simulink model "DFADAS2_SenFus_v1_201204RC_training_210115"  (R2018b)
settings: Solver=FixedStepDiscrete  StartTime=0.0  StopTime=inf  FixedStep=0.002  RelTol=1e-3  EnableMultiTasking=on
PreLoadFcn:
  | RTWConfigurationCB('preloadfcn', bdroot);
libraries: canmsglib x108, simulink x48, canfdmsglib x12
(part 17 of 28)

== system DFADAS2_SenFus_v1_201204RC_training_210115/Signal Input (Input)/Signal Input (50ms) (Input50)/Rear Right Radar(S1) Objects Information (RRRdr)/S0 Data Frame Read/Enabled Subsystem/M4ObjInfo1 ==
  msg : Inport
  MValue : Inport  Port=2
  RemainderCnt : Inport  Port=3
  obj_num : Inport  Port=4
  Add3 : Sum
  Bus Creator1 : BusCreator  Inputs=24
  Bus Creator2 : BusCreator  Inputs=24
  Constant : Constant  Value=9
  Data Type Conversion{,1..3} (4 alike) : DataTypeConversion  OutDataTypeStr=uint16
  Data Type Conversion5 : DataTypeConversion  OutDataTypeStr=int16
  Demux : Demux  Outputs=24
  Demux1 : Demux  Outputs=24
  If : If  NumInputs=3  IfExpression=u1 == 1  ElseIfExpressions=u2 == 0 & u3 == 1  ShowElse=off
  If Action Subsystem1 : Subsystem  TreatAsAtomicUnit=on
  If Action Subsystem2 : Subsystem  TreatAsAtomicUnit=on
  MValueSel : Constant  Value=4
  Memory1 : Memory  InheritSampleTime=on
  Memory2 : Memory  InheritSampleTime=on
  Merge : Merge
  Merge1 : Merge
  Relational Operator : RelationalOperator  Operator===  OutDataTypeStr=boolean  RndMeth=Simplest
  Relational Operator1 : RelationalOperator  Operator=>  OutDataTypeStr=boolean  RndMeth=Simplest
  Subsystem1 : Subsystem
  Subtract : Sum  Inputs=+-
  M40ObjInfo : Outport
  M41ObjInfo : Outport  Port=2
  wires:
  Subsystem1/1(Out) -> Add3/2
  Memory2/1 -> Subsystem1/3(In)
  Data Type Conversion5/1 -> Memory1/1, Subtract/1
  Memory1/1 -> Subtract/2
  RemainderCnt/1 -> Data Type Conversion3/1, Data Type Conversion5/1
  Subtract/1 -> Subsystem1/1(const)
  Constant/1 -> Relational Operator1/2
  obj_num/1 -> Relational Operator1/1
  Relational Operator1/1 -> If Action Subsystem1/3("obj_num ")
  Bus Creator2/1 -> M41ObjInfo/1  "Obj10Info"
  Merge1/1 -> Demux1/1
  Demux1/12 -> Bus Creator2/12  "Orientation_S0_010"
  Demux1/17 -> Bus Creator2/17  "ReferencePoint_S0_010"
  Demux1/22 -> Bus Creator2/22  "YAccStd_S0_010"
  Demux1/23 -> Bus Creator2/23  "YPosStd_S0_010"
  Demux1/8 -> Bus Creator2/8  "XAcc_S0_010"
  Demux1/21 -> Bus Creator2/21  "XVelocityStd_S0_010"
  Demux1/19 -> Bus Creator2/19  "XAccStd_S0_010"
  Demux1/18 -> Bus Creator2/18  "Height_S0_010"
  Demux1/15 -> Bus Creator2/15  "ClassHighest_S0_010"
  Demux1/7 -> Bus Creator2/7  "YVelocity_S0_010"
  Demux1/14 -> Bus Creator2/14  "MovingState_S0_010"
  Demux1/20 -> Bus Creator2/20  "XPosStd_S0_010"
  Demux1/13 -> Bus Creator2/13  "ExistenceProb_S0_010"
  Demux1/9 -> Bus Creator2/9  "YAcc_S0_010"
  Demux1/24 -> Bus Creator2/24  "YVelocityStd_S0_010"
  Demux1/11 -> Bus Creator2/11  "Length_S0_010"
  Demux1/10 -> Bus Creator2/10  "Width_S0_010"
  Demux1/4 -> Bus Creator2/4  "XPos_S0_010"
  Demux1/16 -> Bus Creator2/16  "ClassHighestProb_S0_010"
  Demux1/5 -> Bus Creator2/5  "YPos_S0_010"
  Demux1/3 -> Bus Creator2/3  "ObjMeasured_S0_010"
  Demux1/2 -> Bus Creator2/2  "ObjInit_S0_010"
  Demux1/6 -> Bus Creator2/6  "XVelocity_S0_010"
  Demux1/1 -> Bus Creator2/1  "Id_S0_010"
  Demux/6 -> Bus Creator1/6  "XVelocity_S0_009"
  Demux/1 -> Bus Creator1/1  "Id_S0_009"
  Demux/15 -> Bus Creator1/15  "ClassHighest_S0_009"
  Demux/11 -> Bus Creator1/11  "Length_S0_009"
  Demux/2 -> Bus Creator1/2  "ObjInit_S0_009"
  Demux/8 -> Bus Creator1/8  "XAcc_S0_009"
  Demux/19 -> Bus Creator1/19  "XAccStd_S0_009"
  Demux/4 -> Bus Creator1/4  "XPos_S0_009"
  Demux/21 -> Bus Creator1/21  "XVelocityStd_S0_009"
  Demux/16 -> Bus Creator1/16  "ClassHighestProb_S0_009"
  Demux/3 -> Bus Creator1/3  "ObjMeasured_S0_009"
  Demux/23 -> Bus Creator1/23  "YPosStd_S0_009"
  Demux/5 -> Bus Creator1/5  "YPos_S0_009"
  Demux/14 -> Bus Creator1/14  "MovingState_S0_009"
  Demux/9 -> Bus Creator1/9  "YAcc_S0_009"
  Demux/12 -> Bus Creator1/12  "Orientation_S0_009"
  Demux/18 -> Bus Creator1/18  "Height_S0_009"
  Demux/20 -> Bus Creator1/20  "XPosStd_S0_009"
  Demux/7 -> Bus Creator1/7  "YVelocity_S0_009"
  Demux/22 -> Bus Creator1/22  "YAccStd_S0_009"
  Demux/17 -> Bus Creator1/17  "ReferencePoint_S0_009"
  Demux/13 -> Bus Creator1/13  "ExistenceProb_S0_009"
  Demux/10 -> Bus Creator1/10  "Width_S0_009"
  Demux/24 -> Bus Creator1/24  "YVelocityStd_S0_009"
  Bus Creator1/1 -> M40ObjInfo/1  "Obj9Info"
  Merge/1 -> Demux/1
  Data Type Conversion3/1 -> If/3
  Data Type Conversion2/1 -> If/2
  Data Type Conversion1/1 -> If/1
  If Action Subsystem1/2(M41ObjInfo) -> Merge1/1
  If Action Subsystem2/2(ZeroObjInfo1) -> Merge1/2
  MValueSel/1 -> Relational Operator/1, If Action Subsystem1/2("MValueSel ")
  If Action Subsystem2/1(ZeroObjInfo0) -> Merge/2
  If Action Subsystem1/1(M40ObjInfo) -> Merge/1
  Relational Operator/1 -> Data Type Conversion1/1, Data Type Conversion/1
  If/2 -> If Action Subsystem2/Action
  If/1 -> If Action Subsystem1/Action
  Data Type Conversion/1 -> Add3/1
  Add3/1 -> Data Type Conversion2/1, Memory2/1  "MValueSim"
  MValue/1 -> Relational Operator/2
  msg/1 -> If Action Subsystem1/1(msg)

== system DFADAS2_SenFus_v1_201204RC_training_210115/Signal Input (Input)/Signal Input (50ms) (Input50)/Rear Right Radar(S1) Objects Information (RRRdr)/S0 Data Frame Read/Enabled Subsystem/Unpack ==
  Msg : Inport
  RemainderCnt : Inport  Port=2
  Add : Sum
  Bus Selector : BusSelector  Commented=on  OutputSignals=Obj1Info.Id_S0_001
  Constant : Constant  Value=0
  If : If  IfExpression=u1>0  ElseIfExpressions=u1==0
  If Action Subsystem : Subsystem  TreatAsAtomicUnit=on
  If Action Subsystem1 : Subsystem  TreatAsAtomicUnit=on
  Merge : Merge
  Scope : Scope  Commented=on
  MsgOut : Outport
  MValue : Outport  Port=2
  wires:
  RemainderCnt/1 -> If/1
  Merge/1 -> MValue/1
  Constant/1 -> Add/2
  Bus Selector/1 -> Scope/1  "<Id_S0_001>"
  Add/1 -> Merge/1
  If Action Subsystem1/1(DflMValue) -> Merge/2
  If Action Subsystem/2(MValue) -> Add/1
  If Action Subsystem/1(RLRdrObjInfo) -> MsgOut/1, Bus Selector/1
  If/1 -> If Action Subsystem/Action
  Msg/1 -> If Action Subsystem/1(msg)
  If/2 -> If Action Subsystem1/Action

== system DFADAS2_SenFus_v1_201204RC_training_210115/Signal Input (Input)/Signal Input (50ms) (Input50)/Rear Right Radar(S1) Objects Information (RRRdr)/S0 Data Frame Read/Subsystem/M0ObjInfo ==
  Bus Creator1 : BusCreator  Inputs=24
  Bus Creator2 : BusCreator  Inputs=24
  Constant : Constant  Value=[0 0 0 0 0 0 0 0 0 0 0 0 0 0 0 0 0 0 0 0 0 0 0 0 ]
  Constant1 : Constant  Value=[0 0 0 0 0 0 0 0 0 0 0 0 0 0 0 0 0 0 0 0 0 0 0 0 ]
  Demux : Demux  Outputs=24
  Demux1 : Demux  Outputs=24
  M00ObjInfo : Outport
  M01ObjInfo : Outport  Port=2
  wires:
  Demux1/6 -> Bus Creator2/6  "XVelocity_S0_002"
  Demux1/3 -> Bus Creator2/3  "ObjMeasured_S0_002"
  Demux/22 -> Bus Creator1/22  "YAccStd_S0_001"
  Demux1/18 -> Bus Creator2/18  "Height_S0_002"
  Demux/12 -> Bus Creator1/12  "Orientation_S0_001"
  Demux/8 -> Bus Creator1/8  "XAcc_S0_001"
  Constant/1 -> Demux/1
  Demux/10 -> Bus Creator1/10  "Width_S0_001"
  Demux1/2 -> Bus Creator2/2  "ObjInit_S0_002"
  Bus Creator1/1 -> M00ObjInfo/1
  Demux/17 -> Bus Creator1/17  "ReferencePoint_S0_001"
  Bus Creator2/1 -> M01ObjInfo/1  "Obj2Info"
  Demux1/20 -> Bus Creator2/20  "XPosStd_S0_002"
  Demux1/21 -> Bus Creator2/21  "XVelocityStd_S0_002"
  Demux/23 -> Bus Creator1/23  "YPosStd_S0_001"
  Demux1/4 -> Bus Creator2/4  "XPos_S0_002"
  Demux/9 -> Bus Creator1/9  "YAcc_S0_001"
  Demux1/24 -> Bus Creator2/24  "YVelocityStd_S0_002"
  Demux/3 -> Bus Creator1/3  "ObjMeasured_S0_001"
  Demux/11 -> Bus Creator1/11  "Length_S0_001"
  Demux/14 -> Bus Creator1/14  "MovingState_S0_001"
  Demux1/12 -> Bus Creator2/12  "Orientation_S0_002"
  Demux/6 -> Bus Creator1/6  "XVelocity_S0_001"
  Demux1/7 -> Bus Creator2/7  "YVelocity_S0_002"
  Demux1/13 -> Bus Creator2/13  "ExistenceProb_S0_002"
  Demux/7 -> Bus Creator1/7  "YVelocity_S0_001"
  Demux/2 -> Bus Creator1/2  "ObjInit_S0_001"
  Demux/4 -> Bus Creator1/4  "XPos_S0_001"
  Demux/18 -> Bus Creator1/18  "Height_S0_001"
  Demux/15 -> Bus Creator1/15  "ClassHighest_S0_001"
  Demux/13 -> Bus Creator1/13  "ExistenceProb_S0_001"
  Demux/16 -> Bus Creator1/16  "ClassHighestProb_S0_001"
  Demux/19 -> Bus Creator1/19  "XAccStd_S0_001"
  Demux/24 -> Bus Creator1/24  "YVelocityStd_S0_001"
  Demux1/11 -> Bus Creator2/11  "Length_S0_002"
  Demux1/16 -> Bus Creator2/16  "ClassHighestProb_S0_002"
  Demux1/5 -> Bus Creator2/5  "YPos_S0_002"
  Demux1/14 -> Bus Creator2/14  "MovingState_S0_002"
  Demux1/9 -> Bus Creator2/9  "YAcc_S0_002"
  Demux1/1 -> Bus Creator2/1  "Id_S0_002"
  Constant1/1 -> Demux1/1
  Demux/21 -> Bus Creator1/21  "XVelocityStd_S0_001"
  Demux1/15 -> Bus Creator2/15  "ClassHighest_S0_002"
  Demux1/8 -> Bus Creator2/8  "XAcc_S0_002"
  Demux/5 -> Bus Creator1/5  "YPos_S0_001"
  Demux/20 -> Bus Creator1/20  "XPosStd_S0_001"
  Demux1/19 -> Bus Creator2/19  "XAccStd_S0_002"
  Demux1/22 -> Bus Creator2/22  "YAccStd_S0_002"
  Demux1/10 -> Bus Creator2/10  "Width_S0_002"
  Demux/1 -> Bus Creator1/1  "Id_S0_001"
  Demux1/17 -> Bus Creator2/17  "ReferencePoint_S0_002"
  Demux1/23 -> Bus Creator2/23  "YPosStd_S0_002"

== system DFADAS2_SenFus_v1_201204RC_training_210115/Signal Input (Input)/Signal Input (50ms) (Input50)/Rear Right Radar(S1) Objects Information (RRRdr)/S0 Data Frame Read/Subsystem/M1ObjInfo1 ==
  Bus Creator1 : BusCreator  Inputs=24
  Bus Creator2 : BusCreator  Inputs=24
  Constant : Constant  Value=[0 0 0 0 0 0 0 0 0 0 0 0 0 0 0 0 0 0 0 0 0 0 0 0 ]
  Constant1 : Constant  Value=[0 0 0 0 0 0 0 0 0 0 0 0 0 0 0 0 0 0 0 0 0 0 0 0 ]
  Demux : Demux  Outputs=24
  Demux1 : Demux  Outputs=24
  M10ObjInfo : Outport
  M11ObjInfo : Outport  Port=2
  wires:
  Constant1/1 -> Demux1/1
  Constant/1 -> Demux/1
  Bus Creator1/1 -> M10ObjInfo/1  "Obj3Info"
  Demux/24 -> Bus Creator1/24  "YVelocityStd_S0_003"
  Demux/10 -> Bus Creator1/10  "Width_S0_003"
  Demux/13 -> Bus Creator1/13  "ExistenceProb_S0_003"
  Demux/17 -> Bus Creator1/17  "ReferencePoint_S0_003"
  Demux/22 -> Bus Creator1/22  "YAccStd_S0_003"
  Demux/7 -> Bus Creator1/7  "YVelocity_S0_003"
  Demux/20 -> Bus Creator1/20  "XPosStd_S0_003"
  Demux/18 -> Bus Creator1/18  "Height_S0_003"
  Demux/12 -> Bus Creator1/12  "Orientation_S0_003"
  Demux/9 -> Bus Creator1/9  "YAcc_S0_003"
  Demux/14 -> Bus Creator1/14  "MovingState_S0_003"
  Demux/5 -> Bus Creator1/5  "YPos_S0_003"
  Demux/23 -> Bus Creator1/23  "YPosStd_S0_003"
  Demux/3 -> Bus Creator1/3  "ObjMeasured_S0_003"
  Demux/16 -> Bus Creator1/16  "ClassHighestProb_S0_003"
  Demux/21 -> Bus Creator1/21  "XVelocityStd_S0_003"
  Demux/4 -> Bus Creator1/4  "XPos_S0_003"
  Demux/19 -> Bus Creator1/19  "XAccStd_S0_003"
  Demux/8 -> Bus Creator1/8  "XAcc_S0_003"
  Demux/2 -> Bus Creator1/2  "ObjInit_S0_003"
  Demux/11 -> Bus Creator1/11  "Length_S0_003"
  Demux/15 -> Bus Creator1/15  "ClassHighest_S0_003"
  Demux/1 -> Bus Creator1/1  "Id_S0_003"
  Demux/6 -> Bus Creator1/6  "XVelocity_S0_003"
  Demux1/1 -> Bus Creator2/1  "Id_S0_004"
  Demux1/6 -> Bus Creator2/6  "XVelocity_S0_004"
  Demux1/2 -> Bus Creator2/2  "ObjInit_S0_004"
  Demux1/3 -> Bus Creator2/3  "ObjMeasured_S0_004"
  Demux1/5 -> Bus Creator2/5  "YPos_S0_004"
  Demux1/16 -> Bus Creator2/16  "ClassHighestProb_S0_004"
  Demux1/4 -> Bus Creator2/4  "XPos_S0_004"
  Demux1/10 -> Bus Creator2/10  "Width_S0_004"
  Demux1/11 -> Bus Creator2/11  "Length_S0_004"
  Demux1/24 -> Bus Creator2/24  "YVelocityStd_S0_004"
  Demux1/9 -> Bus Creator2/9  "YAcc_S0_004"
  Demux1/13 -> Bus Creator2/13  "ExistenceProb_S0_004"
  Demux1/20 -> Bus Creator2/20  "XPosStd_S0_004"
  Demux1/14 -> Bus Creator2/14  "MovingState_S0_004"
  Demux1/7 -> Bus Creator2/7  "YVelocity_S0_004"
  Demux1/15 -> Bus Creator2/15  "ClassHighest_S0_004"
  Demux1/18 -> Bus Creator2/18  "Height_S0_004"
  Demux1/19 -> Bus Creator2/19  "XAccStd_S0_004"
  Demux1/21 -> Bus Creator2/21  "XVelocityStd_S0_004"
  Demux1/8 -> Bus Creator2/8  "XAcc_S0_004"
  Demux1/23 -> Bus Creator2/23  "YPosStd_S0_004"
  Demux1/22 -> Bus Creator2/22  "YAccStd_S0_004"
  Demux1/17 -> Bus Creator2/17  "ReferencePoint_S0_004"
  Demux1/12 -> Bus Creator2/12  "Orientation_S0_004"
  Bus Creator2/1 -> M11ObjInfo/1  "Obj4Info"

== system DFADAS2_SenFus_v1_201204RC_training_210115/Signal Input (Input)/Signal Input (50ms) (Input50)/Rear Right Radar(S1) Objects Information (RRRdr)/S0 Data Frame Read/Subsystem/M2ObjInfo ==
  Bus Creator1 : BusCreator  Inputs=24
  Bus Creator2 : BusCreator  Inputs=24
  Constant : Constant  Value=[0 0 0 0 0 0 0 0 0 0 0 0 0 0 0 0 0 0 0 0 0 0 0 0 ]
  Constant1 : Constant  Value=[0 0 0 0 0 0 0 0 0 0 0 0 0 0 0 0 0 0 0 0 0 0 0 0 ]
  Demux : Demux  Outputs=24
  Demux1 : Demux  Outputs=24
  M20ObjInfo : Outport
  M21ObjInfo : Outport  Port=2
  wires:
  Constant1/1 -> Demux1/1
  Bus Creator2/1 -> M21ObjInfo/1  "Obj6Info"
  Demux1/12 -> Bus Creator2/12  "Orientation_S0_006"
  Demux1/17 -> Bus Creator2/17  "ReferencePoint_S0_006"
  Demux1/22 -> Bus Creator2/22  "YAccStd_S0_006"
  Demux1/23 -> Bus Creator2/23  "YPosStd_S0_006"
  Demux1/8 -> Bus Creator2/8  "XAcc_S0_006"
  Demux1/21 -> Bus Creator2/21  "XVelocityStd_S0_006"
  Demux1/19 -> Bus Creator2/19  "XAccStd_S0_006"
  Demux1/18 -> Bus Creator2/18  "Height_S0_006"
  Demux1/15 -> Bus Creator2/15  "ClassHighest_S0_006"
  Demux1/7 -> Bus Creator2/7  "YVelocity_S0_006"
  Demux1/14 -> Bus Creator2/14  "MovingState_S0_006"
  Demux1/20 -> Bus Creator2/20  "XPosStd_S0_006"
  Demux1/13 -> Bus Creator2/13  "ExistenceProb_S0_006"
  Demux1/9 -> Bus Creator2/9  "YAcc_S0_006"
  Demux1/24 -> Bus Creator2/24  "YVelocityStd_S0_006"
  Demux1/11 -> Bus Creator2/11  "Length_S0_006"
  Demux1/10 -> Bus Creator2/10  "Width_S0_006"
  Demux1/4 -> Bus Creator2/4  "XPos_S0_006"
  Demux1/16 -> Bus Creator2/16  "ClassHighestProb_S0_006"
  Demux1/5 -> Bus Creator2/5  "YPos_S0_006"
  Demux1/3 -> Bus Creator2/3  "ObjMeasured_S0_006"
  Demux1/2 -> Bus Creator2/2  "ObjInit_S0_006"
  Demux1/6 -> Bus Creator2/6  "XVelocity_S0_006"
  Demux1/1 -> Bus Creator2/1  "Id_S0_006"
  Demux/6 -> Bus Creator1/6  "XVelocity_S0_005"
  Demux/1 -> Bus Creator1/1  "Id_S0_005"
  Demux/15 -> Bus Creator1/15  "ClassHighest_S0_005"
  Demux/11 -> Bus Creator1/11  "Length_S0_005"
  Demux/2 -> Bus Creator1/2  "ObjInit_S0_005"
  Demux/8 -> Bus Creator1/8  "XAcc_S0_005"
  Demux/19 -> Bus Creator1/19  "XAccStd_S0_005"
  Demux/4 -> Bus Creator1/4  "XPos_S0_005"
  Demux/21 -> Bus Creator1/21  "XVelocityStd_S0_005"
  Demux/16 -> Bus Creator1/16  "ClassHighestProb_S0_005"
  Demux/3 -> Bus Creator1/3  "ObjMeasured_S0_005"
  Demux/23 -> Bus Creator1/23  "YPosStd_S0_005"
  Demux/5 -> Bus Creator1/5  "YPos_S0_005"
  Demux/14 -> Bus Creator1/14  "MovingState_S0_005"
  Demux/9 -> Bus Creator1/9  "YAcc_S0_005"
  Demux/12 -> Bus Creator1/12  "Orientation_S0_005"
  Demux/18 -> Bus Creator1/18  "Height_S0_005"
  Demux/20 -> Bus Creator1/20  "XPosStd_S0_005"
  Demux/7 -> Bus Creator1/7  "YVelocity_S0_005"
  Demux/22 -> Bus Creator1/22  "YAccStd_S0_005"
  Demux/17 -> Bus Creator1/17  "ReferencePoint_S0_005"
  Demux/13 -> Bus Creator1/13  "ExistenceProb_S0_005"
  Demux/10 -> Bus Creator1/10  "Width_S0_005"
  Demux/24 -> Bus Creator1/24  "YVelocityStd_S0_005"
  Bus Creator1/1 -> M20ObjInfo/1  "Obj5Info"
  Constant/1 -> Demux/1

== system DFADAS2_SenFus_v1_201204RC_training_210115/Signal Input (Input)/Signal Input (50ms) (Input50)/Rear Right Radar(S1) Objects Information (RRRdr)/S0 Data Frame Read/Subsystem/M3ObjInfo ==
  Bus Creator1 : BusCreator  Inputs=24
  Bus Creator2 : BusCreator  Inputs=24
  Constant : Constant  Value=[0 0 0 0 0 0 0 0 0 0 0 0 0 0 0 0 0 0 0 0 0 0 0 0 ]
  Constant1 : Constant  Value=[0 0 0 0 0 0 0 0 0 0 0 0 0 0 0 0 0 0 0 0 0 0 0 0 ]
  Demux : Demux  Outputs=24
  Demux1 : Demux  Outputs=24
  M30ObjInfo : Outport
  M31ObjInfo : Outport  Port=2
  wires:
  Constant1/1 -> Demux1/1
  Constant/1 -> Demux/1
  Bus Creator1/1 -> M30ObjInfo/1  "Obj7Info"
  Demux/24 -> Bus Creator1/24  "YVelocityStd_S0_007"
  Demux/10 -> Bus Creator1/10  "Width_S0_007"
  Demux/13 -> Bus Creator1/13  "ExistenceProb_S0_007"
  Demux/17 -> Bus Creator1/17  "ReferencePoint_S0_007"
  Demux/22 -> Bus Creator1/22  "YAccStd_S0_007"
  Demux/7 -> Bus Creator1/7  "YVelocity_S0_007"
  Demux/20 -> Bus Creator1/20  "XPosStd_S0_007"
  Demux/18 -> Bus Creator1/18  "Height_S0_007"
  Demux/12 -> Bus Creator1/12  "Orientation_S0_007"
  Demux/9 -> Bus Creator1/9  "YAcc_S0_007"
  Demux/14 -> Bus Creator1/14  "MovingState_S0_007"
  Demux/5 -> Bus Creator1/5  "YPos_S0_007"
  Demux/23 -> Bus Creator1/23  "YPosStd_S0_007"
  Demux/3 -> Bus Creator1/3  "ObjMeasured_S0_007"
  Demux/16 -> Bus Creator1/16  "ClassHighestProb_S0_007"
  Demux/21 -> Bus Creator1/21  "XVelocityStd_S0_007"
  Demux/4 -> Bus Creator1/4  "XPos_S0_007"
  Demux/19 -> Bus Creator1/19  "XAccStd_S0_007"
  Demux/8 -> Bus Creator1/8  "XAcc_S0_007"
  Demux/2 -> Bus Creator1/2  "ObjInit_S0_007"
  Demux/11 -> Bus Creator1/11  "Length_S0_007"
  Demux/15 -> Bus Creator1/15  "ClassHighest_S0_007"
  Demux/1 -> Bus Creator1/1  "Id_S0_007"
  Demux/6 -> Bus Creator1/6  "XVelocity_S0_007"
  Demux1/1 -> Bus Creator2/1  "Id_S0_008"
  Demux1/6 -> Bus Creator2/6  "XVelocity_S0_008"
  Demux1/2 -> Bus Creator2/2  "ObjInit_S0_008"
  Demux1/3 -> Bus Creator2/3  "ObjMeasured_S0_008"
  Demux1/5 -> Bus Creator2/5  "YPos_S0_008"
  Demux1/16 -> Bus Creator2/16  "ClassHighestProb_S0_008"
  Demux1/4 -> Bus Creator2/4  "XPos_S0_008"
  Demux1/10 -> Bus Creator2/10  "Width_S0_008"
  Demux1/11 -> Bus Creator2/11  "Length_S0_008"
  Demux1/24 -> Bus Creator2/24  "YVelocityStd_S0_008"
  Demux1/9 -> Bus Creator2/9  "YAcc_S0_008"
  Demux1/13 -> Bus Creator2/13  "ExistenceProb_S0_008"
  Demux1/20 -> Bus Creator2/20  "XPosStd_S0_008"
  Demux1/14 -> Bus Creator2/14  "MovingState_S0_008"
  Demux1/7 -> Bus Creator2/7  "YVelocity_S0_008"
  Demux1/15 -> Bus Creator2/15  "ClassHighest_S0_008"
  Demux1/18 -> Bus Creator2/18  "Height_S0_008"
  Demux1/19 -> Bus Creator2/19  "XAccStd_S0_008"
  Demux1/21 -> Bus Creator2/21  "XVelocityStd_S0_008"
  Demux1/8 -> Bus Creator2/8  "XAcc_S0_008"
  Demux1/23 -> Bus Creator2/23  "YPosStd_S0_008"
  Demux1/22 -> Bus Creator2/22  "YAccStd_S0_008"
  Demux1/17 -> Bus Creator2/17  "ReferencePoint_S0_008"
  Demux1/12 -> Bus Creator2/12  "Orientation_S0_008"
  Bus Creator2/1 -> M31ObjInfo/1  "Obj8Info"

== system DFADAS2_SenFus_v1_201204RC_training_210115/Signal Input (Input)/Signal Input (50ms) (Input50)/Rear Right Radar(S1) Objects Information (RRRdr)/S0 Data Frame Read/Subsystem/M4ObjInfo1 ==
  Bus Creator1 : BusCreator  Inputs=24
  Bus Creator2 : BusCreator  Inputs=24
  Constant : Constant  Value=[0 0 0 0 0 0 0 0 0 0 0 0 0 0 0 0 0 0 0 0 0 0 0 0 ]
  Constant1 : Constant  Value=[0 0 0 0 0 0 0 0 0 0 0 0 0 0 0 0 0 0 0 0 0 0 0 0 ]
  Demux : Demux  Outputs=24
  Demux1 : Demux  Outputs=24
  M40ObjInfo : Outport
  M41ObjInfo : Outport  Port=2
  wires:
  Constant1/1 -> Demux1/1
  Constant/1 -> Demux/1
  Bus Creator2/1 -> M41ObjInfo/1  "Obj10Info"
  Demux1/12 -> Bus Creator2/12  "Orientation_S0_010"
  Demux1/17 -> Bus Creator2/17  "ReferencePoint_S0_010"
  Demux1/22 -> Bus Creator2/22  "YAccStd_S0_010"
  Demux1/23 -> Bus Creator2/23  "YPosStd_S0_010"
  Demux1/8 -> Bus Creator2/8  "XAcc_S0_010"
  Demux1/21 -> Bus Creator2/21  "XVelocityStd_S0_010"
  Demux1/19 -> Bus Creator2/19  "XAccStd_S0_010"
  Demux1/18 -> Bus Creator2/18  "Height_S0_010"
  Demux1/15 -> Bus Creator2/15  "ClassHighest_S0_010"
  Demux1/7 -> Bus Creator2/7  "YVelocity_S0_010"
  Demux1/14 -> Bus Creator2/14  "MovingState_S0_010"
  Demux1/20 -> Bus Creator2/20  "XPosStd_S0_010"
  Demux1/13 -> Bus Creator2/13  "ExistenceProb_S0_010"
  Demux1/9 -> Bus Creator2/9  "YAcc_S0_010"
  Demux1/24 -> Bus Creator2/24  "YVelocityStd_S0_010"
  Demux1/11 -> Bus Creator2/11  "Length_S0_010"
  Demux1/10 -> Bus Creator2/10  "Width_S0_010"
  Demux1/4 -> Bus Creator2/4  "XPos_S0_010"
  Demux1/16 -> Bus Creator2/16  "ClassHighestProb_S0_010"
  Demux1/5 -> Bus Creator2/5  "YPos_S0_010"
  Demux1/3 -> Bus Creator2/3  "ObjMeasured_S0_010"
  Demux1/2 -> Bus Creator2/2  "ObjInit_S0_010"
  Demux1/6 -> Bus Creator2/6  "XVelocity_S0_010"
  Demux1/1 -> Bus Creator2/1  "Id_S0_010"
  Demux/6 -> Bus Creator1/6  "XVelocity_S0_009"
  Demux/1 -> Bus Creator1/1  "Id_S0_009"
  Demux/15 -> Bus Creator1/15  "ClassHighest_S0_009"
  Demux/11 -> Bus Creator1/11  "Length_S0_009"
  Demux/2 -> Bus Creator1/2  "ObjInit_S0_009"
  Demux/8 -> Bus Creator1/8  "XAcc_S0_009"
  Demux/19 -> Bus Creator1/19  "XAccStd_S0_009"
  Demux/4 -> Bus Creator1/4  "XPos_S0_009"
  Demux/21 -> Bus Creator1/21  "XVelocityStd_S0_009"
  Demux/16 -> Bus Creator1/16  "ClassHighestProb_S0_009"
  Demux/3 -> Bus Creator1/3  "ObjMeasured_S0_009"
  Demux/23 -> Bus Creator1/23  "YPosStd_S0_009"
  Demux/5 -> Bus Creator1/5  "YPos_S0_009"
  Demux/14 -> Bus Creator1/14  "MovingState_S0_009"
  Demux/9 -> Bus Creator1/9  "YAcc_S0_009"
  Demux/12 -> Bus Creator1/12  "Orientation_S0_009"
  Demux/18 -> Bus Creator1/18  "Height_S0_009"
  Demux/20 -> Bus Creator1/20  "XPosStd_S0_009"
  Demux/7 -> Bus Creator1/7  "YVelocity_S0_009"
  Demux/22 -> Bus Creator1/22  "YAccStd_S0_009"
  Demux/17 -> Bus Creator1/17  "ReferencePoint_S0_009"
  Demux/13 -> Bus Creator1/13  "ExistenceProb_S0_009"
  Demux/10 -> Bus Creator1/10  "Width_S0_009"
  Demux/24 -> Bus Creator1/24  "YVelocityStd_S0_009"
  Bus Creator1/1 -> M40ObjInfo/1  "Obj9Info"

== system DFADAS2_SenFus_v1_201204RC_training_210115/Signal Input (Input)/Signal Input (10ms) (Input10)/VehInfo/Body Electric System State Receive and Processing (BESRx)/Steering Lamp CAN Frame PreProcess (StLampCANFrmPPrcs)/CAN Diagnosis (CANDia)/Break State Diagnosis (BreStDia) ==
  note: Error Flag Discription:
      | 0 : Normal
      | 1 : Fault
  BreStDia_tiCANRxSmplT : Inport
  BreStDia_tiTLim : Inport  Port=2
  BreStDia_cfCANRxNewFlg : Inport  Port=3
  Add : Sum
  Add1 : Sum  Inputs=+-
  Constant : Constant  SampleTime=-1
  Constant1 : Constant  Value=0  SampleTime=-1
  Constant2 : Constant  Value=0  SampleTime=-1
  Constant3 : Constant  SampleTime=-1
  Divide : Product  Inputs=**
  Divide1 : Product  Inputs=/*
  Memory : Memory  InheritSampleTime=on
  Switch : Switch  Criteria=u2 ~= 0
  Switch1 : Switch
  BreStDia_efErrFlg : Outport
  wires:
  Constant1/1 -> Switch/1
  Constant/1 -> Switch/3
  Switch/1 -> Add/1, Divide/2
  Memory/1 -> Add/2
  Divide/1 -> Memory/1
  Add/1 -> Divide/1, Add1/2
  BreStDia_cfCANRxNewFlg/1 -> Switch/2
  BreStDia_tiCANRxSmplT/1 -> Divide1/1
  BreStDia_tiTLim/1 -> Divide1/2
  Add1/1 -> Switch1/2
  Constant2/1 -> Switch1/1
  Constant3/1 -> Switch1/3
  Switch1/1 -> BreStDia_efErrFlg/1
  Divide1/1 -> Add1/1

== system DFADAS2_SenFus_v1_201204RC_training_210115/Signal Input (Input)/Signal Input (10ms) (Input10)/VehInfo/Body Electric System State Receive and Processing (BESRx)/Steering Lamp CAN Frame PreProcess (StLampCANFrmPPrcs)/CAN Diagnosis (CANDia)/CAN Frame DTC Generator (CANFrmDTCGtr) ==
  CANFrmDTCGtr_efBreStDiaErrFlg : Inport
  CANFrmDTCGtr_efChkSumDiaErrFlg : Inport  Port=2
  CANFrmDTCGtr_efRllCntDiaErrFlg : Inport  Port=3

== system DFADAS2_SenFus_v1_201204RC_training_210115/Signal Input (Input)/Signal Input (10ms) (Input10)/VehInfo/Body Electric System State Receive and Processing (BESRx)/Steering Lamp CAN Frame PreProcess (StLampCANFrmPPrcs)/CAN Diagnosis (CANDia)/CheckSum Diagnosis (ChkSumDia) ==
  ChkSumDia_regCANMsgPrev : Inport
  Bit Check(BChk) : Subsystem  TreatAsAtomicUnit=on
  CAN Message Data Extended (CMsgDaX) : S-Function  FunctionName=CANMsg_DataAcq  SFunctionDeploymentMode=off  EnableBusSupport=off
  ChkSumDia_efErrFlg : Outport
  wires:
  Bit Check(BChk)/1(BChk_efErrFlg) -> ChkSumDia_efErrFlg/1
  ChkSumDia_regCANMsgPrev/1 -> CAN Message Data Extended (CMsgDaX)/1
  CAN Message Data Extended (CMsgDaX)/1 -> Bit Check(BChk)/1(BChk_bRawDa)

== system DFADAS2_SenFus_v1_201204RC_training_210115/Signal Input (Input)/Signal Input (10ms) (Input10)/VehInfo/Body Electric System State Receive and Processing (BESRx)/Steering Lamp CAN Frame PreProcess (StLampCANFrmPPrcs)/CAN Diagnosis (CANDia)/RollingCounter Diagnosis (RllCntDia) ==
  note: RollingCounter Error Flag Discription:
      | 1 : Fault
      | 0 : Normal
  RllCntChk_ctRollingCounter : Inport
  Add : Sum  Inputs=+-
  Add1 : Sum  Inputs=+-
  Constant : Constant  OutDataTypeStr=single  SampleTime=-1
  Constant1 : Constant  Value=0  OutDataTypeStr=single  SampleTime=-1
  Constant2 : Constant  Value=-1  OutDataTypeStr=single  SampleTime=-1
  Constant3 : Constant  OutDataTypeStr=single  SampleTime=-1
  Data Type Conversion : DataTypeConversion  OutDataTypeStr=single
  Switch : Switch  Criteria=u2 ~= 0
  Switch1 : Switch  Threshold=14.5
  Unit Delay : UnitDelay  SampleTime=-1
  RllCntChk_efErrorFlag : Outport
  wires:
  RllCntChk_ctRollingCounter/1 -> Data Type Conversion/1
  Add/1 -> Add1/1
  Constant/1 -> Add1/2
  Constant1/1 -> Switch/3
  Constant3/1 -> Switch/1
  Add1/1 -> Switch/2
  Data Type Conversion/1 -> Add/1, Unit Delay/1
  Unit Delay/1 -> Switch1/2, Switch1/3
  Switch1/1 -> Add/2
  Constant2/1 -> Switch1/1
  Switch/1 -> RllCntChk_efErrorFlag/1

== system DFADAS2_SenFus_v1_201204RC_training_210115/Signal Input (Input)/Signal Input (10ms) (Input10)/VehInfo/Function Keys State Receive and Processing (FKeyStRx)/Key Enable CAN Frame PreProcess (KeyEnaCANFrmPPrcs)/CAN Diagnosis (CANDia)/Break State Diagnosis (BreStDia) ==
  note: Error Flag Discription:
      | 0 : Normal
      | 1 : Fault
  BreStDia_tiCANRxSmplT : Inport
  BreStDia_tiTLim : Inport  Port=2
  BreStDia_cfCANRxNewFlg : Inport  Port=3
  Add : Sum
  Add1 : Sum  Inputs=+-
  Constant : Constant  SampleTime=-1
  Constant1 : Constant  Value=0  SampleTime=-1
  Constant2 : Constant  Value=0  SampleTime=-1
  Constant3 : Constant  SampleTime=-1
  Divide : Product  Inputs=**
  Divide1 : Product  Inputs=/*
  Memory : Memory  InheritSampleTime=on
  Switch : Switch  Criteria=u2 ~= 0
  Switch1 : Switch
  BreStDia_efErrFlg : Outport
  wires:
  Divide1/1 -> Add1/1
  Switch1/1 -> BreStDia_efErrFlg/1
  Constant3/1 -> Switch1/3
  Constant2/1 -> Switch1/1
  Add1/1 -> Switch1/2
  BreStDia_tiTLim/1 -> Divide1/2
  BreStDia_tiCANRxSmplT/1 -> Divide1/1
  BreStDia_cfCANRxNewFlg/1 -> Switch/2
  Add/1 -> Add1/2, Divide/1
  Divide/1 -> Memory/1
  Memory/1 -> Add/2
  Switch/1 -> Divide/2, Add/1
  Constant/1 -> Switch/3
  Constant1/1 -> Switch/1

== system DFADAS2_SenFus_v1_201204RC_training_210115/Signal Input (Input)/Signal Input (10ms) (Input10)/VehInfo/Function Keys State Receive and Processing (FKeyStRx)/Key Enable CAN Frame PreProcess (KeyEnaCANFrmPPrcs)/CAN Diagnosis (CANDia)/CAN Frame DTC Generator (CANFrmDTCGtr) ==
  CANFrmDTCGtr_efBreStDiaErrFlg : Inport
  CANFrmDTCGtr_efChkSumDiaErrFlg : Inport  Port=2
  CANFrmDTCGtr_efRllCntDiaErrFlg : Inport  Port=3

== system DFADAS2_SenFus_v1_201204RC_training_210115/Signal Input (Input)/Signal Input (10ms) (Input10)/VehInfo/Function Keys State Receive and Processing (FKeyStRx)/Key Enable CAN Frame PreProcess (KeyEnaCANFrmPPrcs)/CAN Diagnosis (CANDia)/CheckSum Diagnosis (ChkSumDia) ==
  ChkSumDia_regCANMsgPrev : Inport
  Bit Check(BChk) : Subsystem  TreatAsAtomicUnit=on
  CAN Message Data Extended (CMsgDaX) : S-Function  FunctionName=CANMsg_DataAcq  SFunctionDeploymentMode=off  EnableBusSupport=off
  ChkSumDia_efErrFlg : Outport
  wires:
  CAN Message Data Extended (CMsgDaX)/1 -> Bit Check(BChk)/1(BChk_bRawDa)
  ChkSumDia_regCANMsgPrev/1 -> CAN Message Data Extended (CMsgDaX)/1
  Bit Check(BChk)/1(BChk_efErrFlg) -> ChkSumDia_efErrFlg/1

== system DFADAS2_SenFus_v1_201204RC_training_210115/Signal Input (Input)/Signal Input (10ms) (Input10)/VehInfo/Function Keys State Receive and Processing (FKeyStRx)/Key Enable CAN Frame PreProcess (KeyEnaCANFrmPPrcs)/CAN Diagnosis (CANDia)/RollingCounter Diagnosis (RllCntDia) ==
  note: RollingCounter Error Flag Discription:
      | 1 : Fault
      | 0 : Normal
  RllCntChk_ctRollingCounter : Inport
  Add : Sum  Inputs=+-
  Add1 : Sum  Inputs=+-
  Constant : Constant  OutDataTypeStr=single  SampleTime=-1
  Constant1 : Constant  Value=0  OutDataTypeStr=single  SampleTime=-1
  Constant2 : Constant  Value=-1  OutDataTypeStr=single  SampleTime=-1
  Constant3 : Constant  OutDataTypeStr=single  SampleTime=-1
  Data Type Conversion : DataTypeConversion  OutDataTypeStr=single
  Switch : Switch  Criteria=u2 ~= 0
  Switch1 : Switch  Threshold=14.5
  Unit Delay : UnitDelay  SampleTime=-1
  RllCntChk_efErrorFlag : Outport
  wires:
  Switch/1 -> RllCntChk_efErrorFlag/1
  Constant2/1 -> Switch1/1
  Switch1/1 -> Add/2
  Unit Delay/1 -> Switch1/3, Switch1/2
  Data Type Conversion/1 -> Unit Delay/1, Add/1
  Add1/1 -> Switch/2
  Constant3/1 -> Switch/1
  Constant1/1 -> Switch/3
  Constant/1 -> Add1/2
  Add/1 -> Add1/1
  RllCntChk_ctRollingCounter/1 -> Data Type Conversion/1

== system DFADAS2_SenFus_v1_201204RC_training_210115/Signal Input (Input)/Signal Input (10ms) (Input10)/VehInfo/MP5 Signal Receive (MP5Rx)1/CAN Diagnosis (CANDia)/CheckSum Diagnosis (ChkSumDia)/Bit Check(BChk) ==
  note: Bit Check Discription:
      | Byte0: Checksum
      | Byte1-7: Test signal
  BChk_bRawDa : Inport
  Bit Operating (BOp) : Subsystem
  Byte0 : Selector  IndexMode=Zero-based  InputPortWidth=8  IndexOptions=Index vector (dialog)  Indices=0  OutputSizes=1
  Byte1 : Selector  IndexMode=Zero-based  InputPortWidth=8  IndexOptions=Index vector (dialog)  Indices=1  OutputSizes=1
  Byte2 : Selector  IndexMode=Zero-based  InputPortWidth=8  IndexOptions=Index vector (dialog)  Indices=2  OutputSizes=1
  Byte3 : Selector  IndexMode=Zero-based  InputPortWidth=8  IndexOptions=Index vector (dialog)  Indices=3  OutputSizes=1
  Byte4 : Selector  IndexMode=Zero-based  InputPortWidth=8  IndexOptions=Index vector (dialog)  Indices=4  OutputSizes=1
  Byte5 : Selector  IndexMode=Zero-based  InputPortWidth=8  IndexOptions=Index vector (dialog)  Indices=5  OutputSizes=1
  Byte6 : Selector  IndexMode=Zero-based  InputPortWidth=8  IndexOptions=Index vector (dialog)  Indices=6  OutputSizes=1
  Byte7 : Selector  IndexMode=Zero-based  InputPortWidth=8  IndexOptions=Index vector (dialog)  Indices=7  OutputSizes=1
  BChk_efErrFlg : Outport
  wires:
  Byte0/1 -> Bit Operating (BOp)/1(Chksum in Frame)
  Bit Operating (BOp)/1(BOp_efChkSumErrFlg) -> BChk_efErrFlg/1
  Byte7/1 -> Bit Operating (BOp)/8(BOp_bByte7)
  Byte6/1 -> Bit Operating (BOp)/7(BOp_bByte6)
  Byte5/1 -> Bit Operating (BOp)/6(BOp_bByte5)
  Byte4/1 -> Bit Operating (BOp)/5(BOp_bByte4)
  Byte3/1 -> Bit Operating (BOp)/4(BOp_bByte3)
  Byte2/1 -> Bit Operating (BOp)/3(BOp_bByte2)
  Byte1/1 -> Bit Operating (BOp)/2(BOp_bByte1)
  BChk_bRawDa/1 -> Byte7/1, Byte6/1, Byte5/1, Byte4/1, Byte3/1, Byte2/1, Byte1/1, Byte0/1

== system DFADAS2_SenFus_v1_201204RC_training_210115/Signal Input (Input)/Signal Input (10ms) (Input10)/VehInfo/Vehicle Movement Signal Receive and Processing (VehMovRx)/VehSpd CAN Frame PreProcess (VehSpdCANFrmPPrcs)/CAN Diagnosis (CANDia)/Break State Diagnosis (BreStDia) ==
  note: Error Flag Discription:
      | 0 : Normal
      | 1 : Fault
  BreStDia_tiCANRxSmplT : Inport
  BreStDia_tiTLim : Inport  Port=2
  BreStDia_cfCANRxNewFlg : Inport  Port=3
  Add : Sum
  Add1 : Sum  Inputs=+-
  Constant : Constant  SampleTime=-1
  Constant1 : Constant  Value=0  SampleTime=-1
  Constant2 : Constant  Value=0  SampleTime=-1
  Constant3 : Constant  SampleTime=-1
  Divide : Product  Inputs=**
  Divide1 : Product  Inputs=/*
  Memory : Memory  InheritSampleTime=on
  Switch : Switch  Criteria=u2 ~= 0
  Switch1 : Switch
  BreStDia_efErrFlg : Outport
  wires:
  Divide1/1 -> Add1/1
  Switch1/1 -> BreStDia_efErrFlg/1
  Constant3/1 -> Switch1/3
  Constant2/1 -> Switch1/1
  Add1/1 -> Switch1/2
  BreStDia_tiTLim/1 -> Divide1/2
  BreStDia_tiCANRxSmplT/1 -> Divide1/1
  BreStDia_cfCANRxNewFlg/1 -> Switch/2
  Add/1 -> Add1/2, Divide/1
  Divide/1 -> Memory/1
  Memory/1 -> Add/2
  Switch/1 -> Divide/2, Add/1
  Constant/1 -> Switch/3
  Constant1/1 -> Switch/1

== system DFADAS2_SenFus_v1_201204RC_training_210115/Signal Input (Input)/Signal Input (10ms) (Input10)/VehInfo/Vehicle Movement Signal Receive and Processing (VehMovRx)/VehSpd CAN Frame PreProcess (VehSpdCANFrmPPrcs)/CAN Diagnosis (CANDia)/CAN Frame DTC Generator (CANFrmDTCGtr) ==
  CANFrmDTCGtr_efBreStDiaErrFlg : Inport
  CANFrmDTCGtr_efChkSumDiaErrFlg : Inport  Port=2
  CANFrmDTCGtr_efRllCntDiaErrFlg : Inport  Port=3

== system DFADAS2_SenFus_v1_201204RC_training_210115/Signal Input (Input)/Signal Input (10ms) (Input10)/VehInfo/Vehicle Movement Signal Receive and Processing (VehMovRx)/VehSpd CAN Frame PreProcess (VehSpdCANFrmPPrcs)/CAN Diagnosis (CANDia)/CheckSum Diagnosis (ChkSumDia) ==
  ChkSumDia_regCANMsgPrev : Inport
  Bit Check(BChk) : Subsystem  TreatAsAtomicUnit=on
  CAN Message Data Extended (CMsgDaX) : S-Function  FunctionName=CANMsg_DataAcq  SFunctionDeploymentMode=off  EnableBusSupport=off
  ChkSumDia_efErrFlg : Outport
  wires:
  CAN Message Data Extended (CMsgDaX)/1 -> Bit Check(BChk)/1(BChk_bRawDa)
  ChkSumDia_regCANMsgPrev/1 -> CAN Message Data Extended (CMsgDaX)/1
  Bit Check(BChk)/1(BChk_efErrFlg) -> ChkSumDia_efErrFlg/1

== system DFADAS2_SenFus_v1_201204RC_training_210115/Signal Input (Input)/Signal Input (10ms) (Input10)/VehInfo/Vehicle Movement Signal Receive and Processing (VehMovRx)/VehSpd CAN Frame PreProcess (VehSpdCANFrmPPrcs)/CAN Diagnosis (CANDia)/RollingCounter Diagnosis (RllCntDia) ==
  note: RollingCounter Error Flag Discription:
      | 1 : Fault
      | 0 : Normal
  RllCntChk_ctRollingCounter : Inport
  Add : Sum  Inputs=+-
  Add1 : Sum  Inputs=+-
  Constant : Constant  OutDataTypeStr=single  SampleTime=-1
  Constant1 : Constant  Value=0  OutDataTypeStr=single  SampleTime=-1
  Constant2 : Constant  Value=-1  OutDataTypeStr=single  SampleTime=-1
  Constant3 : Constant  OutDataTypeStr=single  SampleTime=-1
  Data Type Conversion : DataTypeConversion  OutDataTypeStr=single
  Switch : Switch  Criteria=u2 ~= 0
  Switch1 : Switch  Threshold=14.5
  Unit Delay : UnitDelay  SampleTime=-1
  RllCntChk_efErrorFlag : Outport
  wires:
  Switch/1 -> RllCntChk_efErrorFlag/1
  Constant2/1 -> Switch1/1
  Switch1/1 -> Add/2
  Unit Delay/1 -> Switch1/3, Switch1/2
  Data Type Conversion/1 -> Unit Delay/1, Add/1
  Add1/1 -> Switch/2
  Constant3/1 -> Switch/1
  Constant1/1 -> Switch/3
  Constant/1 -> Add1/2
  Add/1 -> Add1/1
  RllCntChk_ctRollingCounter/1 -> Data Type Conversion/1

== system DFADAS2_SenFus_v1_201204RC_training_210115/Signal Input (Input)/Signal Input (10ms) (Input10)/VehInfo/Vehicle Movement Signal Receive and Processing (VehMovRx)/Yaw State CAN Frame PreProcess (YawCANFrmPPrcs)/CAN Diagnosis (CANDia)/Break State Diagnosis (BreStDia) ==
  note: Error Flag Discription:
      | 0 : Normal
      | 1 : Fault
  BreStDia_tiCANRxSmplT : Inport
  BreStDia_tiTLim : Inport  Port=2
  BreStDia_cfCANRxNewFlg : Inport  Port=3
  Add : Sum
  Add1 : Sum  Inputs=+-
  Constant : Constant  SampleTime=-1
  Constant1 : Constant  Value=0  SampleTime=-1
  Constant2 : Constant  Value=0  SampleTime=-1
  Constant3 : Constant  SampleTime=-1
  Divide : Product  Inputs=**
  Divide1 : Product  Inputs=/*
  Memory : Memory  InheritSampleTime=on
  Switch : Switch  Criteria=u2 ~= 0
  Switch1 : Switch
  BreStDia_efErrFlg : Outport
  wires:
  Divide1/1 -> Add1/1
  Switch1/1 -> BreStDia_efErrFlg/1
  Constant3/1 -> Switch1/3
  Constant2/1 -> Switch1/1
  Add1/1 -> Switch1/2
  BreStDia_tiTLim/1 -> Divide1/2
  BreStDia_tiCANRxSmplT/1 -> Divide1/1
  BreStDia_cfCANRxNewFlg/1 -> Switch/2
  Add/1 -> Add1/2, Divide/1
  Divide/1 -> Memory/1
  Memory/1 -> Add/2
  Switch/1 -> Divide/2, Add/1
  Constant/1 -> Switch/3
  Constant1/1 -> Switch/1

== system DFADAS2_SenFus_v1_201204RC_training_210115/Signal Input (Input)/Signal Input (10ms) (Input10)/VehInfo/Vehicle Movement Signal Receive and Processing (VehMovRx)/Yaw State CAN Frame PreProcess (YawCANFrmPPrcs)/CAN Diagnosis (CANDia)/CAN Frame DTC Generator (CANFrmDTCGtr) ==
  CANFrmDTCGtr_efBreStDiaErrFlg : Inport
  CANFrmDTCGtr_efChkSumDiaErrFlg : Inport  Port=2
  CANFrmDTCGtr_efRllCntDiaErrFlg : Inport  Port=3

== system DFADAS2_SenFus_v1_201204RC_training_210115/Signal Input (Input)/Signal Input (10ms) (Input10)/VehInfo/Vehicle Movement Signal Receive and Processing (VehMovRx)/Yaw State CAN Frame PreProcess (YawCANFrmPPrcs)/CAN Diagnosis (CANDia)/CheckSum Diagnosis (ChkSumDia) ==
  ChkSumDia_regCANMsgPrev : Inport
  Bit Check(BChk) : Subsystem  TreatAsAtomicUnit=on
  CAN Message Data Extended (CMsgDaX) : S-Function  FunctionName=CANMsg_DataAcq  SFunctionDeploymentMode=off  EnableBusSupport=off
  ChkSumDia_efErrFlg : Outport
  wires:
  CAN Message Data Extended (CMsgDaX)/1 -> Bit Check(BChk)/1(BChk_bRawDa)
  ChkSumDia_regCANMsgPrev/1 -> CAN Message Data Extended (CMsgDaX)/1
  Bit Check(BChk)/1(BChk_efErrFlg) -> ChkSumDia_efErrFlg/1

== system DFADAS2_SenFus_v1_201204RC_training_210115/Signal Input (Input)/Signal Input (10ms) (Input10)/VehInfo/Vehicle Movement Signal Receive and Processing (VehMovRx)/Yaw State CAN Frame PreProcess (YawCANFrmPPrcs)/CAN Diagnosis (CANDia)/RollingCounter Diagnosis (RllCntDia) ==
  note: RollingCounter Error Flag Discription:
      | 1 : Fault
      | 0 : Normal
  RllCntChk_ctRollingCounter : Inport
  Add : Sum  Inputs=+-
  Add1 : Sum  Inputs=+-
  Constant : Constant  OutDataTypeStr=single  SampleTime=-1
  Constant1 : Constant  Value=0  OutDataTypeStr=single  SampleTime=-1
  Constant2 : Constant  Value=-1  OutDataTypeStr=single  SampleTime=-1
  Constant3 : Constant  OutDataTypeStr=single  SampleTime=-1
  Data Type Conversion : DataTypeConversion  OutDataTypeStr=single
  Switch : Switch  Criteria=u2 ~= 0
  Switch1 : Switch  Threshold=14.5
  Unit Delay : UnitDelay  SampleTime=-1
  RllCntChk_efErrorFlag : Outport
  wires:
  Switch/1 -> RllCntChk_efErrorFlag/1
  Constant2/1 -> Switch1/1
  Switch1/1 -> Add/2
  Unit Delay/1 -> Switch1/3, Switch1/2
  Data Type Conversion/1 -> Unit Delay/1, Add/1
  Add1/1 -> Switch/2
  Constant3/1 -> Switch/1
  Constant1/1 -> Switch/3
  Constant/1 -> Add1/2
  Add/1 -> Add1/1
  RllCntChk_ctRollingCounter/1 -> Data Type Conversion/1

== system DFADAS2_SenFus_v1_201204RC_training_210115/Signal Input (Input)/Signal Input (50ms) (Input50)/Cmr/CmrInfo/L0 Information (L0Info) /CAN Diagnosis (CANDia)1/Break State Diagnosis (BreStDia) ==
  note: Error Flag Discription:
      | 0 : Normal
      | 1 : Fault
  BreStDia_tiCANRxSmplT : Inport
  BreStDia_tiTLim : Inport  Port=2
  BreStDia_cfCANRxNewFlg : Inport  Port=3
  Add : Sum
  Add1 : Sum  Inputs=+-
  Constant : Constant  SampleTime=-1
  Constant1 : Constant  Value=0  SampleTime=-1
  Constant2 : Constant  Value=0  SampleTime=-1
  Constant3 : Constant  SampleTime=-1
  Divide : Product  Inputs=**
  Divide1 : Product  Inputs=/*
  Memory : Memory  InheritSampleTime=on
  Switch : Switch  Criteria=u2 ~= 0
  Switch1 : Switch
  BreStDia_efErrFlg : Outport
  wires:
  Divide1/1 -> Add1/1
  Switch1/1 -> BreStDia_efErrFlg/1
  Constant3/1 -> Switch1/3
  Constant2/1 -> Switch1/1
  Add1/1 -> Switch1/2
  BreStDia_tiTLim/1 -> Divide1/2
  BreStDia_tiCANRxSmplT/1 -> Divide1/1
  BreStDia_cfCANRxNewFlg/1 -> Switch/2
  Add/1 -> Add1/2, Divide/1
  Divide/1 -> Memory/1
  Memory/1 -> Add/2
  Switch/1 -> Divide/2, Add/1
  Constant/1 -> Switch/3
  Constant1/1 -> Switch/1

== system DFADAS2_SenFus_v1_201204RC_training_210115/Signal Input (Input)/Signal Input (50ms) (Input50)/Cmr/CmrInfo/L0 Information (L0Info) /CAN Diagnosis (CANDia)1/CAN Frame DTC Generator (CANFrmDTCGtr) ==
  CANFrmDTCGtr_efBreStDiaErrFlg : Inport
  CANFrmDTCGtr_efChkSumDiaErrFlg : Inport  Port=2
  CANFrmDTCGtr_efRllCntDiaErrFlg : Inport  Port=3

== system DFADAS2_SenFus_v1_201204RC_training_210115/Signal Input (Input)/Signal Input (50ms) (Input50)/Cmr/CmrInfo/L0 Information (L0Info) /CAN Diagnosis (CANDia)1/CheckSum Diagnosis (ChkSumDia) ==
  ChkSumDia_regCANMsgPrev : Inport
  Bit Check(BChk) : Subsystem  TreatAsAtomicUnit=on
      settings: RTWSystemCode=Nonreusable function
  CAN Message Data Extended (CMsgDaX) : S-Function  FunctionName=CANMsg_DataAcq  SFunctionDeploymentMode=off  EnableBusSupport=off  mask(CANMsg_DataExt){}
      mask help: This block extracts the raw data from the data field of the input CAN frame signal and outputs it as a 1-D array of data type uint8.
      mask Display:
      | color('blue');text(0.98,0.9,'NovSteeds','horizontalAlignment','right');color('black');text(0.5,0.5,'CAN Message\nData Extraction','horizontalAlignment','center');
      | port_label('input',1,'CAN_Msg');
      | port_label('output',1,'RawData');
  ChkSumDia_efErrFlg : Outport
  wires:
  CAN Message Data Extended (CMsgDaX)/1 -> Bit Check(BChk)/1(BChk_bRawDa)
  ChkSumDia_regCANMsgPrev/1 -> CAN Message Data Extended (CMsgDaX)/1
  Bit Check(BChk)/1(BChk_efErrFlg) -> ChkSumDia_efErrFlg/1

== system DFADAS2_SenFus_v1_201204RC_training_210115/Signal Input (Input)/Signal Input (50ms) (Input50)/Cmr/CmrInfo/L0 Information (L0Info) /CAN Diagnosis (CANDia)1/RollingCounter Diagnosis (RllCntDia) ==
  note: RollingCounter Error Flag Discription:
      | 1 : Fault
      | 0 : Normal
  RllCntChk_ctRollingCounter : Inport
  Add : Sum  Inputs=+-
  Add1 : Sum  Inputs=+-
  Constant : Constant  OutDataTypeStr=single  SampleTime=-1
  Constant1 : Constant  Value=0  OutDataTypeStr=single  SampleTime=-1
  Constant2 : Constant  Value=-1  OutDataTypeStr=single  SampleTime=-1
  Constant3 : Constant  OutDataTypeStr=single  SampleTime=-1
  Data Type Conversion : DataTypeConversion  OutDataTypeStr=single
  Switch : Switch  Criteria=u2 ~= 0
  Switch1 : Switch  Threshold=14.5
  Unit Delay : UnitDelay  SampleTime=-1
  RllCntChk_efErrorFlag : Outport
  wires:
  Switch/1 -> RllCntChk_efErrorFlag/1
  Constant2/1 -> Switch1/1
  Switch1/1 -> Add/2
  Unit Delay/1 -> Switch1/3, Switch1/2
  Data Type Conversion/1 -> Unit Delay/1, Add/1
  Add1/1 -> Switch/2
  Constant3/1 -> Switch/1
  Constant1/1 -> Switch/3
  Constant/1 -> Add1/2
  Add/1 -> Add1/1
  RllCntChk_ctRollingCounter/1 -> Data Type Conversion/1

== system DFADAS2_SenFus_v1_201204RC_training_210115/Signal Input (Input)/Signal Input (50ms) (Input50)/Cmr/CmrInfo/L1 Information (L1Info)/CAN Diagnosis (CANDia)/Break State Diagnosis (BreStDia) ==
  note: Error Flag Discription:
      | 0 : Normal
      | 1 : Fault
  BreStDia_tiCANRxSmplT : Inport
  BreStDia_tiTLim : Inport  Port=2
  BreStDia_cfCANRxNewFlg : Inport  Port=3
  Add : Sum
  Add1 : Sum  Inputs=+-
  Constant : Constant  SampleTime=-1
  Constant1 : Constant  Value=0  SampleTime=-1
  Constant2 : Constant  Value=0  SampleTime=-1
  Constant3 : Constant  SampleTime=-1
  Divide : Product  Inputs=**
  Divide1 : Product  Inputs=/*
  Memory : Memory  InheritSampleTime=on
  Switch : Switch  Criteria=u2 ~= 0
  Switch1 : Switch
  BreStDia_efErrFlg : Outport
  wires:
  Divide1/1 -> Add1/1
  Switch1/1 -> BreStDia_efErrFlg/1
  Constant3/1 -> Switch1/3
  Constant2/1 -> Switch1/1
  Add1/1 -> Switch1/2
  BreStDia_tiTLim/1 -> Divide1/2
  BreStDia_tiCANRxSmplT/1 -> Divide1/1
  BreStDia_cfCANRxNewFlg/1 -> Switch/2
  Add/1 -> Add1/2, Divide/1
  Divide/1 -> Memory/1
  Memory/1 -> Add/2
  Switch/1 -> Divide/2, Add/1
  Constant/1 -> Switch/3
  Constant1/1 -> Switch/1

== system DFADAS2_SenFus_v1_201204RC_training_210115/Signal Input (Input)/Signal Input (50ms) (Input50)/Cmr/CmrInfo/L1 Information (L1Info)/CAN Diagnosis (CANDia)/CAN Frame DTC Generator (CANFrmDTCGtr) ==
  CANFrmDTCGtr_efBreStDiaErrFlg : Inport
  CANFrmDTCGtr_efChkSumDiaErrFlg : Inport  Port=2
  CANFrmDTCGtr_efRllCntDiaErrFlg : Inport  Port=3

== system DFADAS2_SenFus_v1_201204RC_training_210115/Signal Input (Input)/Signal Input (50ms) (Input50)/Cmr/CmrInfo/L1 Information (L1Info)/CAN Diagnosis (CANDia)/CheckSum Diagnosis (ChkSumDia) ==
  ChkSumDia_regCANMsgPrev : Inport
  Bit Check(BChk) : Subsystem  TreatAsAtomicUnit=on
      settings: RTWSystemCode=Nonreusable function
  CAN Message Data Extended (CMsgDaX) : S-Function  FunctionName=CANMsg_DataAcq  SFunctionDeploymentMode=off  EnableBusSupport=off  mask(CANMsg_DataExt){}
      mask help: This block extracts the raw data from the data field of the input CAN frame signal and outputs it as a 1-D array of data type uint8.
      mask Display:
      | color('blue');text(0.98,0.9,'NovSteeds','horizontalAlignment','right');color('black');text(0.5,0.5,'CAN Message\nData Extraction','horizontalAlignment','center');
      | port_label('input',1,'CAN_Msg');
      | port_label('output',1,'RawData');
  ChkSumDia_efErrFlg : Outport
  wires:
  CAN Message Data Extended (CMsgDaX)/1 -> Bit Check(BChk)/1(BChk_bRawDa)
  ChkSumDia_regCANMsgPrev/1 -> CAN Message Data Extended (CMsgDaX)/1
  Bit Check(BChk)/1(BChk_efErrFlg) -> ChkSumDia_efErrFlg/1

== system DFADAS2_SenFus_v1_201204RC_training_210115/Signal Input (Input)/Signal Input (50ms) (Input50)/Cmr/CmrInfo/L1 Information (L1Info)/CAN Diagnosis (CANDia)/RollingCounter Diagnosis (RllCntDia) ==
  note: RollingCounter Error Flag Discription:
      | 1 : Fault
      | 0 : Normal
  RllCntChk_ctRollingCounter : Inport
  Add : Sum  Inputs=+-
  Add1 : Sum  Inputs=+-
  Constant : Constant  OutDataTypeStr=single  SampleTime=-1
  Constant1 : Constant  Value=0  OutDataTypeStr=single  SampleTime=-1
  Constant2 : Constant  Value=-1  OutDataTypeStr=single  SampleTime=-1
  Constant3 : Constant  OutDataTypeStr=single  SampleTime=-1
  Data Type Conversion : DataTypeConversion  OutDataTypeStr=single
  Switch : Switch  Criteria=u2 ~= 0
  Switch1 : Switch  Threshold=14.5
  Unit Delay : UnitDelay  SampleTime=-1
  RllCntChk_efErrorFlag : Outport
  wires:
  Switch/1 -> RllCntChk_efErrorFlag/1
  Constant2/1 -> Switch1/1
  Switch1/1 -> Add/2
  Unit Delay/1 -> Switch1/3, Switch1/2
  Data Type Conversion/1 -> Unit Delay/1, Add/1
  Add1/1 -> Switch/2
  Constant3/1 -> Switch/1
  Constant1/1 -> Switch/3
  Constant/1 -> Add1/2
  Add/1 -> Add1/1
  RllCntChk_ctRollingCounter/1 -> Data Type Conversion/1

== system DFADAS2_SenFus_v1_201204RC_training_210115/Signal Input (Input)/Signal Input (50ms) (Input50)/Cmr/CmrInfo/R0 Information (R0Info)/CAN Diagnosis (CANDia)/Break State Diagnosis (BreStDia) ==
  note: Error Flag Discription:
      | 0 : Normal
      | 1 : Fault
  BreStDia_tiCANRxSmplT : Inport
  BreStDia_tiTLim : Inport  Port=2
  BreStDia_cfCANRxNewFlg : Inport  Port=3
  Add : Sum
  Add1 : Sum  Inputs=+-
  Constant : Constant  SampleTime=-1
  Constant1 : Constant  Value=0  SampleTime=-1
  Constant2 : Constant  Value=0  SampleTime=-1
  Constant3 : Constant  SampleTime=-1
  Divide : Product  Inputs=**
  Divide1 : Product  Inputs=/*
  Memory : Memory  InheritSampleTime=on
  Switch : Switch  Criteria=u2 ~= 0
  Switch1 : Switch
  BreStDia_efErrFlg : Outport
  wires:
  Divide1/1 -> Add1/1
  Switch1/1 -> BreStDia_efErrFlg/1
  Constant3/1 -> Switch1/3
  Constant2/1 -> Switch1/1
  Add1/1 -> Switch1/2
  BreStDia_tiTLim/1 -> Divide1/2
  BreStDia_tiCANRxSmplT/1 -> Divide1/1
  BreStDia_cfCANRxNewFlg/1 -> Switch/2
  Add/1 -> Add1/2, Divide/1
  Divide/1 -> Memory/1
  Memory/1 -> Add/2
  Switch/1 -> Divide/2, Add/1
  Constant/1 -> Switch/3
  Constant1/1 -> Switch/1

== system DFADAS2_SenFus_v1_201204RC_training_210115/Signal Input (Input)/Signal Input (50ms) (Input50)/Cmr/CmrInfo/R0 Information (R0Info)/CAN Diagnosis (CANDia)/CAN Frame DTC Generator (CANFrmDTCGtr) ==
  CANFrmDTCGtr_efBreStDiaErrFlg : Inport
  CANFrmDTCGtr_efChkSumDiaErrFlg : Inport  Port=2
  CANFrmDTCGtr_efRllCntDiaErrFlg : Inport  Port=3

== system DFADAS2_SenFus_v1_201204RC_training_210115/Signal Input (Input)/Signal Input (50ms) (Input50)/Cmr/CmrInfo/R0 Information (R0Info)/CAN Diagnosis (CANDia)/CheckSum Diagnosis (ChkSumDia) ==
  ChkSumDia_regCANMsgPrev : Inport
  Bit Check(BChk) : Subsystem  TreatAsAtomicUnit=on
      settings: RTWSystemCode=Nonreusable function
  CAN Message Data Extended (CMsgDaX) : S-Function  FunctionName=CANMsg_DataAcq  SFunctionDeploymentMode=off  EnableBusSupport=off  mask(CANMsg_DataExt){}
      mask help: This block extracts the raw data from the data field of the input CAN frame signal and outputs it as a 1-D array of data type uint8.
      mask Display:
      | color('blue');text(0.98,0.9,'NovSteeds','horizontalAlignment','right');color('black');text(0.5,0.5,'CAN Message\nData Extraction','horizontalAlignment','center');
      | port_label('input',1,'CAN_Msg');
      | port_label('output',1,'RawData');
  ChkSumDia_efErrFlg : Outport
  wires:
  CAN Message Data Extended (CMsgDaX)/1 -> Bit Check(BChk)/1(BChk_bRawDa)
  ChkSumDia_regCANMsgPrev/1 -> CAN Message Data Extended (CMsgDaX)/1
  Bit Check(BChk)/1(BChk_efErrFlg) -> ChkSumDia_efErrFlg/1
